simulink model "simulink_s1_old_version"  (R2020a)
settings: Solver=VariableStepAuto  StartTime=0.0  StopTime=11.25  RelTol=1e-3
values from neighbouring files (symbols this model uses):
  OUT = [t; zeros(1, length(t))]'    [labo1.m]    (also in labo1_estimation_param.m = [t; output]'; simulation_validation.m = [t; output(1000:end)]')
  REF = mean(input(1:300))    [graph_lineariter.m]    (also in labo1.m = 1.5*ones(2,2); labo1_estimation_param.m = mean(input(1:100)); lineariter.m; simulation_validation.m = mean(input(1:1000))*ones(2,2))
settings Model: Creator=Admin  LastModifiedBy=lab04
settings DebuggingCC: UnconnectedInputMsg=none  UnconnectedOutputMsg=none  UnconnectedLineMsg=none
settings ModelReferenceCC: EnableRefExpFcnMdlSchedulingChecks=off
settings RTWCC: Description=Generic Real-Time Target

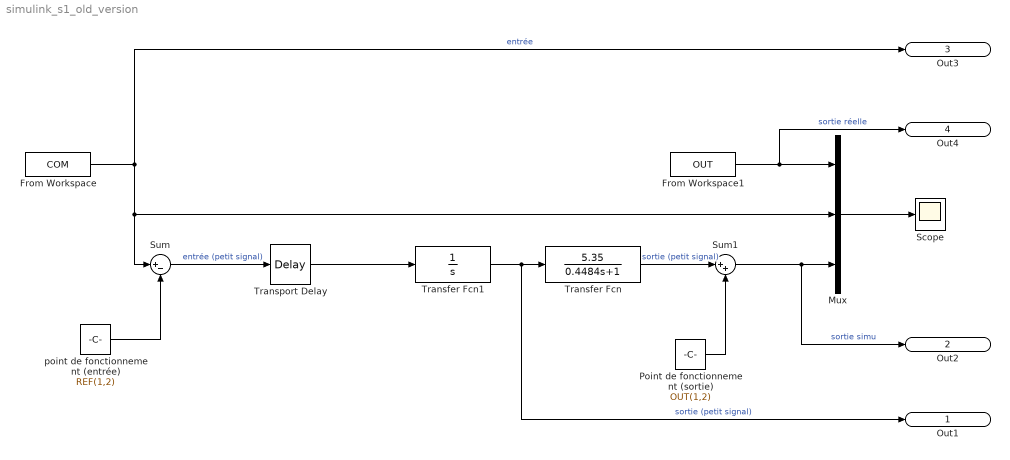
== system simulink_s1_old_version ==
  From Workspace : FromWorkspace  VariableName=COM
  From Workspace1 : FromWorkspace  VariableName=OUT
  Mux : Mux  Inputs=3
  Point de fonctionnement (sortie) : Constant  Value=OUT(1,2)
  Scope : Scope
  Sum : Sum  Inputs=|+-
  Sum1 : Sum  Inputs=|++
  Transfer Fcn : TransferFcn  Numerator=[5.35]  Denominator=[ 0.4484 1 ]
  Transfer Fcn1 : TransferFcn  Denominator="[ 1  0]"
  Transport Delay : TransportDelay  DelayTime=0
  point de fonctionnement (entrée) : Constant  Value=REF(1,2)
  Out1 : Outport  SignalName=step_input
  Out2 : Outport  Port=2  SignalName=simu_output
  Out3 : Outport  Port=3  SignalName=Input
  Out4 : Outport  Port=4  SignalName=sortie réelle
  wires:
  Sum/1 -> Transport Delay/1  "entrée (petit signal)"
  From Workspace1/1 -> Out4/1, Mux/1  "sortie réelle"
  From Workspace/1 -> Sum/1, Mux/2, Out3/1  "entrée"
  Transfer Fcn/1 -> Sum1/1  "sortie (petit signal)"
  Mux/1 -> Scope/1
  Point de fonctionnement (sortie)/1 -> Sum1/2
  point de fonctionnement (entrée)/1 -> Sum/2
  Sum1/1 -> Out2/1, Mux/3  "sortie simu"
  Transfer Fcn1/1 -> Out1/1, Transfer Fcn/1  "sortie (petit signal)"
  Transport Delay/1 -> Transfer Fcn1/1
